simulink model "LQR_ob2"  (R2022b)
settings: Solver=FixedStepAuto  StartTime=0  StopTime=Tf  FixedStep=dt  RelTol=1e-3
values from neighbouring files (symbols this model uses):
  A = [0 1 0 0; -(k1+k2)/m1 -(c1+c2)/m1 k2/m1 c2/m1;0 0 0 1;k2/m2 c2/m2 -k2/m2 -c2/m2]    [LQR_Kalman.m]
  B = [0 0;1/m1 0;0 0;0 1/m2]    [LQR_Kalman.m]
  C = [1 0 0 0;0 0 1 0]    [LQR_Kalman.m]
  c1 = 1    [LQR_Kalman.m]
  c2 = 2    [LQR_Kalman.m]
  control_on = true    [LQR_Kalman.m]
  control_period = 0.01    [LQR_Kalman.m]
  estimation_period = 0.01    [LQR_Kalman.m]
  idealFB_on = false    [LQR_Kalman.m]
  K = inv(R)*B'*P    [LQR_Kalman.m]
  k1 = 10    [LQR_Kalman.m]
  k2 = 20    [LQR_Kalman.m]
  m1 = 1    [LQR_Kalman.m]
  m2 = 5    [LQR_Kalman.m]
  noise_on = false    [LQR_Kalman.m]
  Q_kal = 1e-2    (= 0.01)    [LQR_Kalman.m]
  r = [0 0 0 0]'    [LQR_Kalman.m]
  R_kal = 1e-2    (= 0.01)    [LQR_Kalman.m]
  v1 = 0    [LQR_Kalman.m]
  v2 = 0    [LQR_Kalman.m]
  x1 = 1    [LQR_Kalman.m]
  x2 = 2    [LQR_Kalman.m]
libraries: simulink x2
settings Model: Creator=murayama  LastModifiedBy=ytnpc2021d
settings DataIOCC: SaveFormat=StructureWithTime  ReturnWorkspaceOutputs=off
settings OptimizationCC: BlockReduction=off  BufferReuse=off
settings DebuggingCC: AlgebraicLoopMsg=none

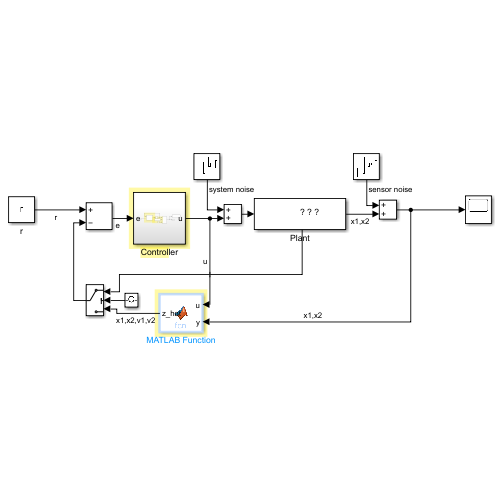
[thumbnail: Simulink's stored preview of the top-level diagram]
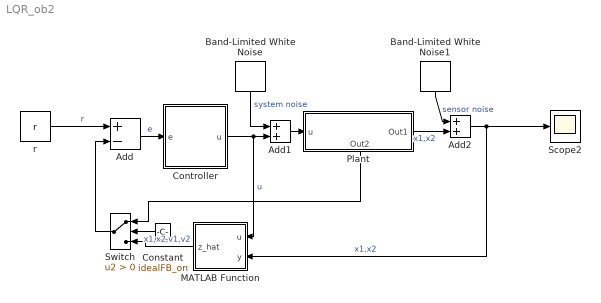
== system LQR_ob2 ==
  Add : Sum  Inputs=+-
  Add1 : Sum
  Add2 : Sum
  Band-Limited White Noise : simulink/Sources/Band-Limited White Noise  Cov=Q_kal*estimation_period*noise_on  Ts=estimation_period  seed=[23341]
  Band-Limited White Noise1 : simulink/Sources/Band-Limited White Noise  Cov=R_kal*estimation_period*noise_on  Ts=estimation_period  seed=[22221]
  Constant : Constant  Value=idealFB_on
  Controller : Subsystem
  MATLAB Function : MATLAB Function  TreatAsAtomicUnit=on
  Plant : Subsystem
      settings: PortSchema="{\"entries\":[{\"content\":{\"sides\":[{\"content\":{\"connectorIds\":[\"In1\"]},\"type\":\"ConnectorPlacement.EquallySpacedRectSide\",\"uuid\":\"f5aa32b0-a431-4113-9166-9a8278ba2da6\"},{\"content\":{\"connectorIds\":[\"Out1\"],\"side\":\"RIGHT\"},\"type\":\"ConnectorPlacement.EquallySpacedRectSide\",\"uuid\":\"0c7c3cb4-750d-40dd-9a30-75948d9fbe92\"},{\"content\":{\"connectorIds\":[],\"side\":\"TOP\"},\"type\":\"ConnectorPlacement.EquallySpacedRectSide\",\"uuid\":\"b05b80b2-958c-441e-9126-94f14a828cf8\"},{\"content\":{\"connectorIds\":[\"Out2\"],\"side\":\"BOTTOM\"},\"type\":\"ConnectorPlacement.EquallySpacedRectSide\",\"uuid\":\"03e2d5f9-7ce1-44d5-b4d9-17cca3a1f8ae\"}]},\"type\":\"ConnectorPlacement.EquallySpacedConnector\",\"uuid\":\"faaf508f-423b-4aab-b951-b31981e4a857\"}],\"packageUris\":[\"http://schema.mathworks.com/mf0/Connector/R2020b\"],\"version\":\"1.0\"}"
      mask Display: image('C:\Users\murayama\Pictures\バネマスダンパ.png'); % 変更するには、ツールストリップの [イメージの編集] を使用してください。
  Scope2 : Scope
  Switch : Switch  Criteria=u2 > Threshold  SaturateOnIntegerOverflow=off  InputSameDT=off
  r : Constant  Value=r  VectorParams1D=off
  wires:
  r/1 -> Add/1  "r"
  Add/1 -> Controller/1(e)  "e"
  Controller/1(u) -> MATLAB Function/1(u), Add1/2  "u"
  MATLAB Function/1(z_hat) -> Switch/3  "x1,x2,v1,v2"
  Add1/1 -> Plant/1(u)
  Plant/1(Out1) -> Add2/2  "x1,x2"
  Add2/1 -> MATLAB Function/2(y), Scope2/1  "x1,x2"
  Band-Limited White Noise1/1 -> Add2/1  "sensor noise"
  Band-Limited White Noise/1 -> Add1/1  "system noise"
  Plant/2(Out2) -> Switch/1
  Switch/1 -> Add/2
  Constant/1 -> Switch/2

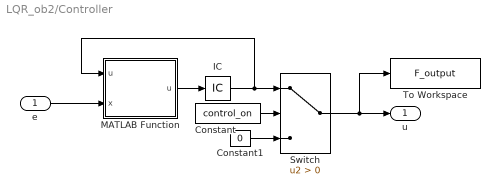
== system LQR_ob2/Controller ==
  e : Inport
  Constant : Constant  Value=control_on
  Constant1 : Constant  Value=0
  IC : InitialCondition  Value=[0 0]'
  MATLAB Function : MATLAB Function  TreatAsAtomicUnit=on
  Switch : Switch  Criteria=u2 > Threshold  SaturateOnIntegerOverflow=off  InputSameDT=off
  To Workspace : ToWorkspace  VariableName=F_output  SaveFormat=Timeseries  SampleTime=-1
  u : Outport
  wires:
  e/1 -> MATLAB Function/2(x)
  Switch/1 -> To Workspace/1, u/1
  Constant/1 -> Switch/2
  Constant1/1 -> Switch/3
  MATLAB Function/1(u) -> IC/1
  IC/1 -> MATLAB Function/1("u "), Switch/1

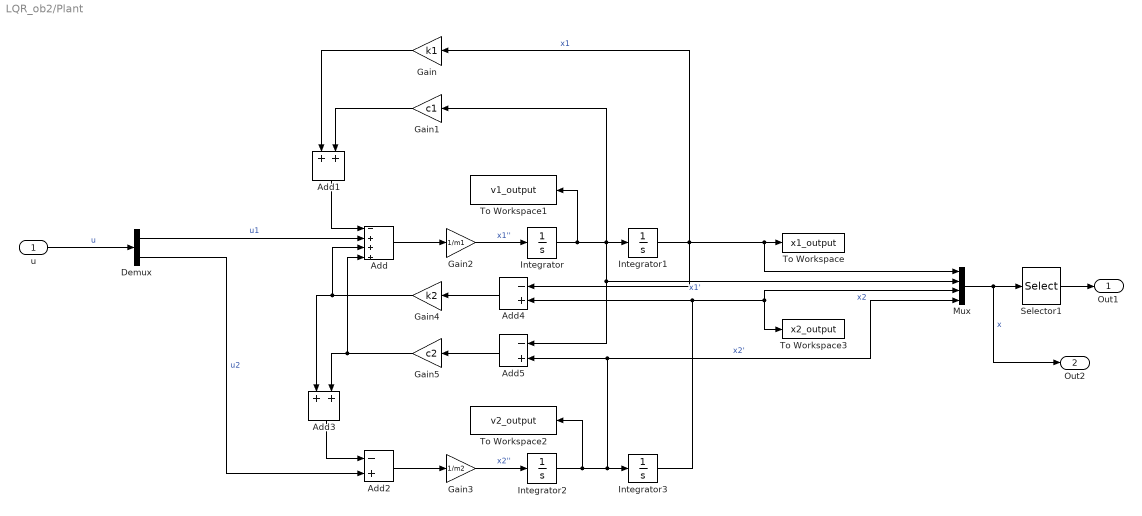
== system LQR_ob2/Plant ==
  u : Inport
  Add : Sum  Inputs=-+++
  Add1 : Sum
  Add2 : Sum  Inputs=-+
  Add3 : Sum
  Add4 : Sum  Inputs=-+
  Add5 : Sum  Inputs=-+
  Demux : Demux  Outputs=2
  Gain : Gain  Gain=k1
  Gain1 : Gain  Gain=c1
  Gain2 : Gain  Gain=1/m1
  Gain3 : Gain  Gain=1/m2
  Gain4 : Gain  Gain=k2
  Gain5 : Gain  Gain=c2
  Integrator : Integrator  InitialCondition=v1
  Integrator1 : Integrator  InitialCondition=x1
  Integrator2 : Integrator  InitialCondition=v2
  Integrator3 : Integrator  InitialCondition=x2
  Mux : Mux
  Selector1 : Selector  InputPortWidth=4  IndexOptions=Index vector (dialog)  Indices=[1 3]  OutputSizes=1
  To Workspace : ToWorkspace  VariableName=x1_output  SaveFormat=Timeseries  SampleTime=-1
  To Workspace1 : ToWorkspace  VariableName=v1_output  SaveFormat=Timeseries  SampleTime=-1
  To Workspace2 : ToWorkspace  VariableName=v2_output  SaveFormat=Timeseries  SampleTime=-1
  To Workspace3 : ToWorkspace  VariableName=x2_output  SaveFormat=Timeseries  SampleTime=-1
  Out1 : Outport
  Out2 : Outport  Port=2
  wires:
  Integrator1/1 -> To Workspace/1, Mux/1, Gain/1, Add4/1  "x1"
  Add1/1 -> Add/1
  Gain/1 -> Add1/1
  Add/1 -> Gain2/1
  Gain2/1 -> Integrator/1  "x1''"
  Integrator/1 -> Add5/1, Mux/2, Gain1/1, Integrator1/1, To Workspace1/1  "x1'"
  Gain1/1 -> Add1/2
  Add2/1 -> Gain3/1
  Gain3/1 -> Integrator2/1  "x2''"
  Integrator2/1 -> To Workspace2/1, Mux/4, Add5/2, Integrator3/1  "x2'"
  Integrator3/1 -> Mux/3, To Workspace3/1, Add4/2  "x2"
  Gain4/1 -> Add3/1, Add/3
  Gain5/1 -> Add/4, Add3/2
  Add3/1 -> Add2/1
  Add4/1 -> Gain4/1
  Add5/1 -> Gain5/1
  Demux/2 -> Add2/2  "u2"
  Demux/1 -> Add/2  "u1"
  u/1 -> Demux/1  "u"
  Mux/1 -> Out2/1, Selector1/1  "x"
  Selector1/1 -> Out1/1

== matlab function LQR_ob2/MATLAB Function ==
  data: u input; z_hat output; y input; A parameter; B parameter; C parameter; estimation_period parameter
function z_hat = fcn(u,y,A, B, C,estimation_period)
dt = estimation_period; %control_period
z1 = z;        b1 = dt*(A*z1+B+h*(y-C*z));
z2 = z+b1/2;   b2 = dt*(A*z2+B*u+h*(y-C*z));
z3 = z+b2/2;   b3 = dt*(A*z3+B*u+h*(y-C*z));
z4 = z+b3;     b4 = dt*(A*z4+B*u+h*(y-C*z));
z = z+(b1+2*b2+2*b3+b4)/6;
z_hat = z;

== matlab function LQR_ob2/Controller/MATLAB Function ==
  data: u input; x input; u output; K parameter; A parameter; B parameter; control_period parameter
function u = fcn(u,x, K, A, B, control_period)
%% 4th Runge-Kutta method
dt = control_period; %control_period
x1 = x;        b1 = dt*(A*x1+B*u);
x2 = x+b1/2;   b2 = dt*(A*x2+B*u);
x3 = x+b2/2;   b3 = dt*(A*x3+B*u);
x4 = x+b3;     b4 = dt*(A*x4+B*u);
x = x+(b1+2*b2+2*b3+b4)/6;
u = K*x;
end
